simulink model "clik_phi_inverse"  (R2022b)
settings: Solver=VariableStepAuto  StartTime=0.0  StopTime=4.0  RelTol=1e-3
undefined symbols (not defined in the file or in its folder): DiscIntNeverNeededParam, q0, Tc
settings Model: Creator=josh7  LastModifiedBy=reube
settings SolverCC: AlgebraicLoopSolver=TrustRegion
settings DebuggingCC: UnconnectedInputMsg=warning  UnconnectedOutputMsg=warning  UnconnectedLineMsg=warning  SFMachineParentedDataDiag=warning  ArithmeticOperatorsInVariantConditions=warning
settings ModelReferenceCC: EnableRefExpFcnMdlSchedulingChecks=on
settings SFSimCC: CustomCodeUndefinedFunction=UseInterfaceOnly

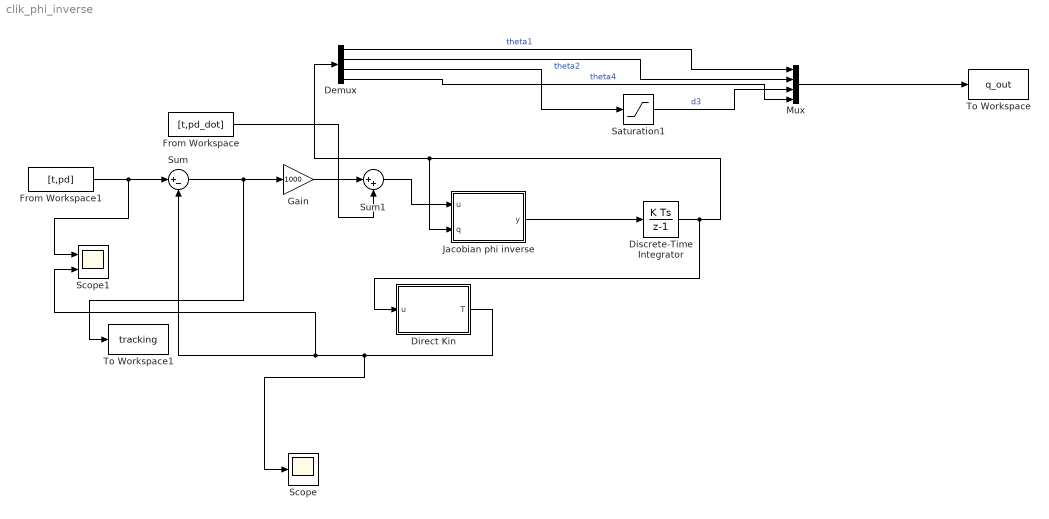
== system clik_phi_inverse ==
  Demux : Demux
  Direct Kin : MATLAB Function  TreatAsAtomicUnit=on
  Discrete-Time Integrator : DiscreteIntegrator  InitialCondition=q0  SampleTime=Tc  LimitOutput=on  UpperSaturationLimit=[pi/2;pi/4;1;2*pi]  LowerSaturationLimit=[-pi/2;-pi/2;0.25;-2*pi]  ICPrevOutput=DiscIntNeverNeededParam  ICPrevScaledInput=DiscIntNeverNeededParam
  From Workspace : FromWorkspace  VariableName=[t,pd_dot]  SampleTime=Tc
  From Workspace1 : FromWorkspace  VariableName=[t,pd]  SampleTime=Tc
  Gain : Gain  Gain=1000
  Jacobian phi inverse : MATLAB Function  TreatAsAtomicUnit=on
  Mux : Mux
  Saturation1 : Saturate  UpperLimit=1  LowerLimit=0.25
  Scope : Scope
  Scope1 : Scope  NumInputPorts=2
  Sum : Sum  Inputs=|+-
  Sum1 : Sum  Inputs=|++
  To Workspace : ToWorkspace  VariableName=q_out  SampleTime=-1
  To Workspace1 : ToWorkspace  VariableName=tracking  SampleTime=Tc
  wires:
  Sum1/1 -> Jacobian phi inverse/1(u)
  Direct Kin/1(T) -> Scope/1, Scope1/2, Sum/2
  Sum/1 -> To Workspace1/1, Gain/1
  From Workspace1/1 -> Scope1/1, Sum/1
  From Workspace/1 -> Sum1/2
  Gain/1 -> Sum1/1
  Jacobian phi inverse/1(y) -> Discrete-Time Integrator/1
  Discrete-Time Integrator/1 -> Direct Kin/1(u), Demux/1, Jacobian phi inverse/2(q)
  Demux/1 -> Mux/1  "theta1"
  Demux/2 -> Mux/2  "theta2"
  Demux/4 -> Mux/4  "theta4"
  Demux/3 -> Saturation1/1
  Saturation1/1 -> Mux/3  "d3"
  Mux/1 -> To Workspace/1

== matlab function clik_phi_inverse/Jacobian phi inverse ==
  data: u input; y output; q input
function y = fcn(u,q)

a1 = 0.5;
a2 = 0.5;

%cos (theta1)
c1 = cos(q(1));
%sin (theta1)
s1 = sin(q(1));
%cos(theta1 + theta2)
c12 = cos(q(1)+q(2));
%sin(theta1 + theta2)
s12 = sin(q(1)+q(2));






JI = [-a2*s12-a1*s1    -a2*s12   0  0; 
            a2*c12+a1*c1      a2*c12   0  0; 
                  0             0      1  0; 
              ];

Q = JI.';
R = Q * inv(JI*Q);
l = R * u;

S = [1 0 0 0; 0 1 0 0; 0 0 1 0; 0 0 0 1] - (R * JI);

K=10;

q0_dot=K * [(-q(1)/(4*(pi)^2));(-4/(9*(pi)^2))*(q(2)+(pi*8));(0.625-q(3))/2.25;-q(4)/(16*(pi)^2)];

y = l + (S * q0_dot);
end

== matlab function clik_phi_inverse/Direct Kin ==
  data: u input; T output
function T = fcn(u)
c1 = cos(u(1));
%Sin(theta1)
s1 = sin(u(1));
%Cos(theta1 + theta2)
c12 = cos(u(1) + u(2));
%Sin(theta1 + theta2)
s12 = sin(u(1) + u(2));
T=[0.5*c12+0.5*c1;
    0.5*s12+0.5*s1;
    u(3)];
